simulink model "bp_check_ver1_3"  (R2020b)
settings: Solver=VariableStepAuto  StartTime=0.0  StopTime=20  RelTol=1e-3
undefined symbols (not defined in the file): sigbuilder_block
libraries: simulink x22
settings Model: Creator=HP  LastModifiedBy=HP

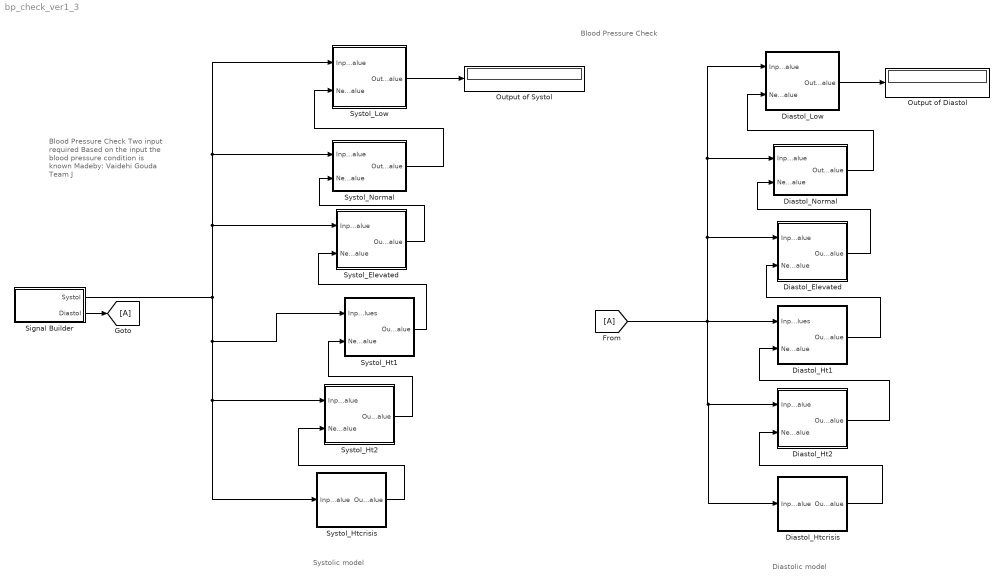
== system bp_check_ver1_3 ==
  note: Systolic model
  note: Blood Pressure Check
      |
      | Two input required
      | Based on the input the blood pressure condition is known
      |
      | Madeby: Vaidehi Gouda
      | Team J
  note: Blood Pressure Check
  note: Diastolic model
  Diastol_Elevated : Subsystem
  Diastol_Ht1 : Subsystem
  Diastol_Ht2 : Subsystem
  Diastol_Htcrisis : Subsystem
  Diastol_Low : Subsystem
  Diastol_Normal : Subsystem
  Output of Diastol : Display
  Output of Systol : Display
  Signal Builder : Subsystem  Tag=STV Subsys  LoadFcn=sigbuilder_block('load');  StartFcn=sigbuilder_block('start');  StopFcn=sigbuilder_block('stop');  ClipboardFcn=sigbuilder_block('clipboard');  mask(Sigbuilder block){tuvar=[0:10]}
      mask help: Simulink:masks:SigbuilderBlock_MD
      mask init:
      | if ~strcmp(get_param(bdroot(gcbh),'SimulationStatus'),'stopped') tuvar = sigbuilder_block('maskInit'); end
      settings: CopyFcn=sigbuilder_block('copy');  DeleteFcn=sigbuilder_block('delete');  ModelCloseFcn=sigbuilder_block('modelClose');  PreSaveFcn=sigbuilder_block('preSave');  PauseFcn=sigbuilder_block('pause');  ContinueFcn=sigbuilder_block('continue');  NameChangeFcn=sigbuilder_block('namechange');  OpenFcn=sigbuilder_block('open',[5.4 30 1141.2 522.6 ]);  CloseFcn=sigbuilder_block('close');
      mask Display: plot(0, 0, 100, 100,[2, 2, 32, 32, 2], [68, 8, 8, 68, 68],[32, 2], [38, 38], [32, 19, 2],[53, 60, 44], [32, 17, 17, 2],[16, 16, 31, 31]);txt = getActiveGroup(gcbh);text(2, 100, txt,'verticalAlignment', 'top');
  Systol_Elevated : Subsystem
  Systol_Ht1 : Subsystem
  Systol_Ht2 : Subsystem
  Systol_Htcrisis : Subsystem
  Systol_Low : Subsystem
  Systol_Normal : Subsystem
  wires:
  Systol_Normal/1(Output_value) -> Systol_Low/2(Next Input value)
  Systol_Elevated/1(Output_value) -> Systol_Normal/2(Next Input value)
  Systol_Ht1/1(Output_value) -> Systol_Elevated/2(Next Input value)
  Systol_Ht2/1(Output_value) -> Systol_Ht1/2(Next Input value)
  Systol_Htcrisis/1(Output_value) -> Systol_Ht2/2(Next Input value)
  Diastol_Htcrisis/1(Output value) -> Diastol_Ht2/2(Next Input value)
  Diastol_Ht2/1(Output_value) -> Diastol_Ht1/2(Next Input value)
  Diastol_Ht1/1(Output_value) -> Diastol_Elevated/2(Next Input value)
  Diastol_Elevated/1(Output value) -> Diastol_Normal/2(Next Input value)
  Diastol_Normal/1(Output_value) -> Diastol_Low/2(Next Input value)
  Diastol_Low/1(Output_value) -> Output of Diastol/1
  Signal Builder/1(Systol) -> Systol_Htcrisis/1(Input value), Systol_Ht2/1(Input value), Systol_Ht1/1(Input values), Systol_Elevated/1(Input value), Systol_Normal/1(Input value), Systol_Low/1(Input_value)
  Systol_Low/1(Output_value) -> Output of Systol/1
  [A] -> Diastol_Elevated/1(Input value), Diastol_Normal/1(Input value), Diastol_Low/1(Input_value), Diastol_Htcrisis/1(Input value), Diastol_Ht2/1(Input value), Diastol_Ht1/1(Input values)
  Signal Builder/2(Diastol) -> [A]

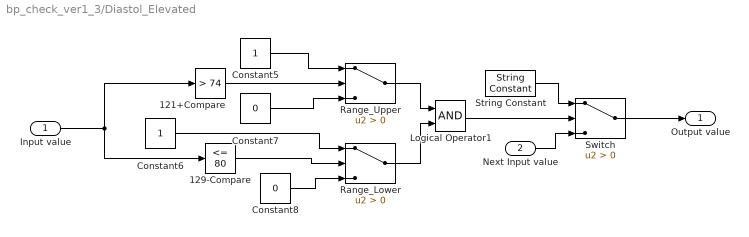
== system bp_check_ver1_3/Diastol_Elevated ==
  Input value : Inport
  Next Input value : Inport  Port=2
  121+Compare : simulink/Logic and Bit Operations/Compare To Constant  relop=>  const=74  OutDataTypeStr=boolean
  129-Compare : simulink/Logic and Bit Operations/Compare To Constant  relop=<=  const=80  OutDataTypeStr=boolean
  Constant5 : Constant
  Constant6 : Constant
  Constant7 : Constant  Value=0
  Constant8 : Constant  Value=0
  Logical Operator1 : Logic  AllPortsSameDT=off  OutDataTypeStr=boolean
  Range_Lower : Switch  Criteria=u2 > Threshold
  Range_Upper : Switch  Criteria=u2 > Threshold
  String Constant : StringConstant  String="\"Eleveted\""
  Switch : Switch  Criteria=u2 > Threshold
  Output value : Outport
  wires:
  Constant7/1 -> Range_Upper/3
  Input value/1 -> 129-Compare/1, 121+Compare/1
  Constant6/1 -> Range_Lower/1
  Constant8/1 -> Range_Lower/3
  Constant5/1 -> Range_Upper/1
  121+Compare/1 -> Range_Upper/2
  Range_Upper/1 -> Logical Operator1/1
  129-Compare/1 -> Range_Lower/2
  Range_Lower/1 -> Logical Operator1/2
  String Constant/1 -> Switch/1
  Logical Operator1/1 -> Switch/2
  Switch/1 -> Output value/1
  Next Input value/1 -> Switch/3

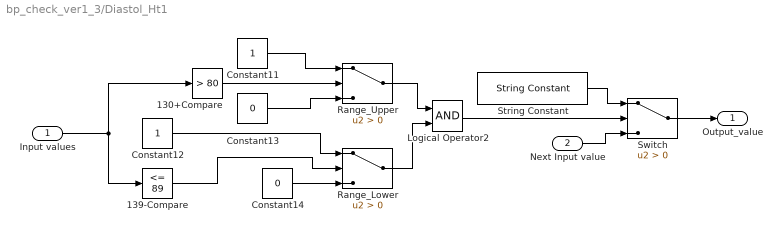
== system bp_check_ver1_3/Diastol_Ht1 ==
  Input values : Inport
  Next Input value : Inport  Port=2
  130+Compare : simulink/Logic and Bit Operations/Compare To Constant  relop=>  const=80  OutDataTypeStr=boolean
  139-Compare : simulink/Logic and Bit Operations/Compare To Constant  relop=<=  const=89  OutDataTypeStr=boolean
  Constant11 : Constant
  Constant12 : Constant
  Constant13 : Constant  Value=0
  Constant14 : Constant  Value=0
  Logical Operator2 : Logic  AllPortsSameDT=off  OutDataTypeStr=boolean
  Range_Lower : Switch  Criteria=u2 > Threshold
  Range_Upper : Switch  Criteria=u2 > Threshold
  String Constant : StringConstant  String="\"Hypertension Stage1\""
  Switch : Switch  Criteria=u2 > Threshold
  Output_value : Outport
  wires:
  Constant13/1 -> Range_Upper/3
  Range_Upper/1 -> Logical Operator2/1
  Range_Lower/1 -> Logical Operator2/2
  139-Compare/1 -> Range_Lower/2
  130+Compare/1 -> Range_Upper/2
  Constant12/1 -> Range_Lower/1
  Constant14/1 -> Range_Lower/3
  Constant11/1 -> Range_Upper/1
  Input values/1 -> 139-Compare/1, 130+Compare/1
  String Constant/1 -> Switch/1
  Logical Operator2/1 -> Switch/2
  Switch/1 -> Output_value/1
  Next Input value/1 -> Switch/3

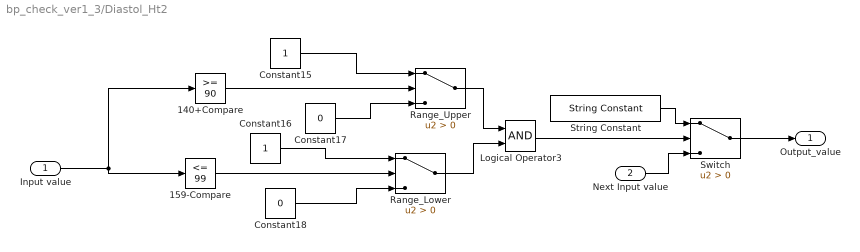
== system bp_check_ver1_3/Diastol_Ht2 ==
  Input value : Inport
  Next Input value : Inport  Port=2
  140+Compare : simulink/Logic and Bit Operations/Compare To Constant  relop=>=  const=90  OutDataTypeStr=boolean
  159-Compare : simulink/Logic and Bit Operations/Compare To Constant  relop=<=  const=99  OutDataTypeStr=boolean
  Constant15 : Constant
  Constant16 : Constant
  Constant17 : Constant  Value=0
  Constant18 : Constant  Value=0
  Logical Operator3 : Logic  AllPortsSameDT=off  OutDataTypeStr=boolean
  Range_Lower : Switch  Criteria=u2 > Threshold
  Range_Upper : Switch  Criteria=u2 > Threshold
  String Constant : StringConstant  String="\"Hypertension Stage2\""
  Switch : Switch  Criteria=u2 > Threshold
  Output_value : Outport
  wires:
  Constant15/1 -> Range_Upper/1
  140+Compare/1 -> Range_Upper/2
  Constant18/1 -> Range_Lower/3
  Range_Lower/1 -> Logical Operator3/2
  Range_Upper/1 -> Logical Operator3/1
  Input value/1 -> 159-Compare/1, 140+Compare/1
  Constant17/1 -> Range_Upper/3
  159-Compare/1 -> Range_Lower/2
  Constant16/1 -> Range_Lower/1
  String Constant/1 -> Switch/1
  Logical Operator3/1 -> Switch/2
  Switch/1 -> Output_value/1
  Next Input value/1 -> Switch/3

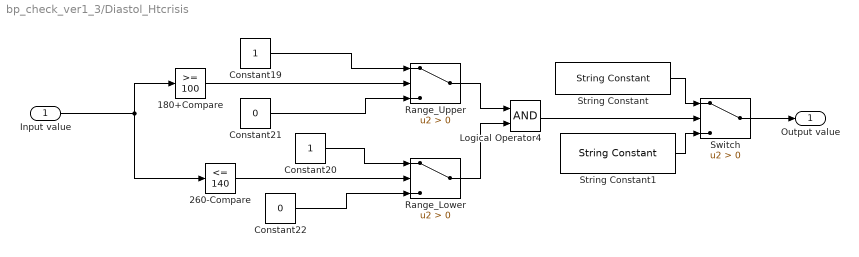
== system bp_check_ver1_3/Diastol_Htcrisis ==
  Input value : Inport
  180+Compare : simulink/Logic and Bit Operations/Compare To Constant  relop=>=  const=100  OutDataTypeStr=boolean
  260-Compare : simulink/Logic and Bit Operations/Compare To Constant  relop=<=  const=140  OutDataTypeStr=boolean
  Constant19 : Constant
  Constant20 : Constant
  Constant21 : Constant  Value=0
  Constant22 : Constant  Value=0
  Logical Operator4 : Logic  AllPortsSameDT=off  OutDataTypeStr=boolean
  Range_Lower : Switch  Criteria=u2 > Threshold
  Range_Upper : Switch  Criteria=u2 > Threshold
  String Constant : StringConstant  String="\"Hypertension crisis\""
  String Constant1 : StringConstant  String="\"Input value not in range\""
  Switch : Switch  Criteria=u2 > Threshold
  Output value : Outport
  wires:
  Input value/1 -> 260-Compare/1, 180+Compare/1
  Constant19/1 -> Range_Upper/1
  Range_Upper/1 -> Logical Operator4/1
  Constant20/1 -> Range_Lower/1
  180+Compare/1 -> Range_Upper/2
  260-Compare/1 -> Range_Lower/2
  Constant22/1 -> Range_Lower/3
  Constant21/1 -> Range_Upper/3
  Range_Lower/1 -> Logical Operator4/2
  String Constant/1 -> Switch/1
  Logical Operator4/1 -> Switch/2
  Switch/1 -> Output value/1
  String Constant1/1 -> Switch/3

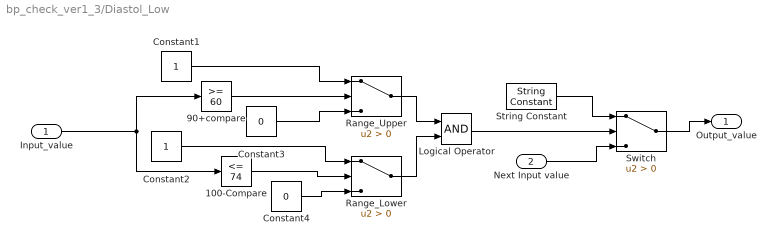
== system bp_check_ver1_3/Diastol_Low ==
  Input_value : Inport
  Next Input value : Inport  Port=2
  100-Compare : simulink/Logic and Bit Operations/Compare To Constant  relop=<=  const=74  OutDataTypeStr=boolean
  90+compare : simulink/Logic and Bit Operations/Compare To Constant  relop=>=  const=60  OutDataTypeStr=boolean
  Constant1 : Constant
  Constant2 : Constant
  Constant3 : Constant  Value=0
  Constant4 : Constant  Value=0
  Logical Operator : Logic  AllPortsSameDT=off  OutDataTypeStr=boolean
  Range_Lower : Switch  Criteria=u2 > Threshold
  Range_Upper : Switch  Criteria=u2 > Threshold
  String Constant : StringConstant  String="\"Low\""
  Switch : Switch  Criteria=u2 > Threshold
  Output_value : Outport
  wires:
  Constant2/1 -> Range_Lower/1
  Constant4/1 -> Range_Lower/3
  90+compare/1 -> Range_Upper/2
  100-Compare/1 -> Range_Lower/2
  Range_Upper/1 -> Logical Operator/1
  Constant1/1 -> Range_Upper/1
  Range_Lower/1 -> Logical Operator/2
  Input_value/1 -> 90+compare/1, 100-Compare/1
  Constant3/1 -> Range_Upper/3
  String Constant/1 -> Switch/1
  Logical Operator/1 -> Switch/2
  Switch/1 -> Output_value/1
  Next Input value/1 -> Switch/3

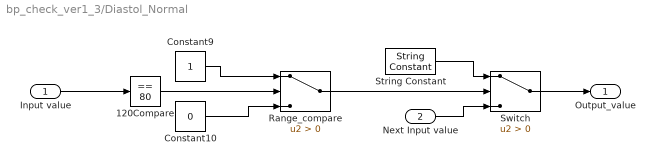
== system bp_check_ver1_3/Diastol_Normal ==
  Input value : Inport
  Next Input value : Inport  Port=2
  120Compare : simulink/Logic and Bit Operations/Compare To Constant  relop===  const=80  OutDataTypeStr=boolean
  Constant10 : Constant  Value=0
  Constant9 : Constant
  Range_compare : Switch  Criteria=u2 > Threshold
  String Constant : StringConstant  String="\"Normal\""
  Switch : Switch  Criteria=u2 > Threshold
  Output_value : Outport
  wires:
  Constant10/1 -> Range_compare/3
  Input value/1 -> 120Compare/1
  120Compare/1 -> Range_compare/2
  Constant9/1 -> Range_compare/1
  String Constant/1 -> Switch/1
  Range_compare/1 -> Switch/2
  Switch/1 -> Output_value/1
  Next Input value/1 -> Switch/3

== system bp_check_ver1_3/Signal Builder ==
  Demux : Demux  Tag=STV Demux  Outputs=2
      settings: DisplayOption=none
  FromWs : FromWorkspace  Tag=STV FromWs  VariableName=tuvar
      SigBuilderData=|
      | common.afterFinalStr = 'Extrapolate'
      | common.sampleTime = 0
      | dataSet.timeRange = [0 2]
      | dataSet.name = 'Sheet1'
      | sbobj.Name = 'Signal Builder'
      | sbobj.Groups.Name = 'Sheet1'
      | sbobj.Groups.Signals(1).Name = 'Systol'
      | sbobj.Groups.Signals(1).XData = [0 0.1 0.2 0.3 0.4 0.5 0.6 0.7 0.8 0.9 1 1.1 1.2 1.3 1.4 1.5 1.6 1.7 1.8 1.9 2]
      | sbobj.Groups.Signals(1).YData = [91 145 132 130 136 140 156 180 95 100 105 102 148 196 142 158 136 135 129 96 109]
      | sbobj.Groups.Signals(2).Name = 'Diastol'
      | sbobj.Groups.Signals(2).XData = [0 0.1 0.2 0.3 0.4 0.5 0.6 0.7 0.8 0.9 1 1.1 1.2 1.3 1.4 1.5 1.6 1.7 1.8 1.9 2]
      | sbobj.Groups.Signals(2).YData = [60 97 84 89 84 90 97 127 67 64 65 64 94 135 98 99 82 84 76 63 70]
      | sbobj.Groups.TimeRange = [0 2]
  Systol : Outport  Tag=STV Outport
  Diastol : Outport  Tag=STV Outport  Port=2
  wires:
  Demux/1 -> Systol/1
  FromWs/1 -> Demux/1
  Demux/2 -> Diastol/1

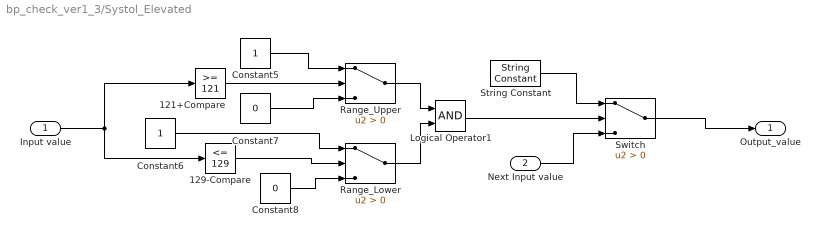
== system bp_check_ver1_3/Systol_Elevated ==
  Input value : Inport
  Next Input value : Inport  Port=2
  121+Compare : simulink/Logic and Bit Operations/Compare To Constant  relop=>=  const=121  OutDataTypeStr=boolean
  129-Compare : simulink/Logic and Bit Operations/Compare To Constant  relop=<=  const=129  OutDataTypeStr=boolean
  Constant5 : Constant
  Constant6 : Constant
  Constant7 : Constant  Value=0
  Constant8 : Constant  Value=0
  Logical Operator1 : Logic  AllPortsSameDT=off  OutDataTypeStr=boolean
  Range_Lower : Switch  Criteria=u2 > Threshold
  Range_Upper : Switch  Criteria=u2 > Threshold
  String Constant : StringConstant  String="\"Elevated\""
  Switch : Switch  Criteria=u2 > Threshold
  Output_value : Outport
  wires:
  Range_Lower/1 -> Logical Operator1/2
  129-Compare/1 -> Range_Lower/2
  Range_Upper/1 -> Logical Operator1/1
  121+Compare/1 -> Range_Upper/2
  Constant5/1 -> Range_Upper/1
  Constant8/1 -> Range_Lower/3
  Constant6/1 -> Range_Lower/1
  Input value/1 -> 121+Compare/1, 129-Compare/1
  Constant7/1 -> Range_Upper/3
  String Constant/1 -> Switch/1
  Logical Operator1/1 -> Switch/2
  Switch/1 -> Output_value/1
  Next Input value/1 -> Switch/3

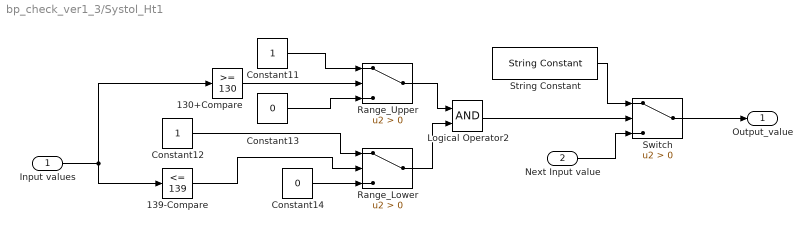
== system bp_check_ver1_3/Systol_Ht1 ==
  Input values : Inport
  Next Input value : Inport  Port=2
  130+Compare : simulink/Logic and Bit Operations/Compare To Constant  relop=>=  const=130  OutDataTypeStr=boolean
  139-Compare : simulink/Logic and Bit Operations/Compare To Constant  relop=<=  const=139  OutDataTypeStr=boolean
  Constant11 : Constant
  Constant12 : Constant
  Constant13 : Constant  Value=0
  Constant14 : Constant  Value=0
  Logical Operator2 : Logic  AllPortsSameDT=off  OutDataTypeStr=boolean
  Range_Lower : Switch  Criteria=u2 > Threshold
  Range_Upper : Switch  Criteria=u2 > Threshold
  String Constant : StringConstant  String="\"Hypertension Stage1\""
  Switch : Switch  Criteria=u2 > Threshold
  Output_value : Outport
  wires:
  Input values/1 -> 139-Compare/1, 130+Compare/1
  Constant11/1 -> Range_Upper/1
  Constant14/1 -> Range_Lower/3
  Constant12/1 -> Range_Lower/1
  130+Compare/1 -> Range_Upper/2
  139-Compare/1 -> Range_Lower/2
  Range_Lower/1 -> Logical Operator2/2
  Range_Upper/1 -> Logical Operator2/1
  Constant13/1 -> Range_Upper/3
  String Constant/1 -> Switch/1
  Logical Operator2/1 -> Switch/2
  Switch/1 -> Output_value/1
  Next Input value/1 -> Switch/3

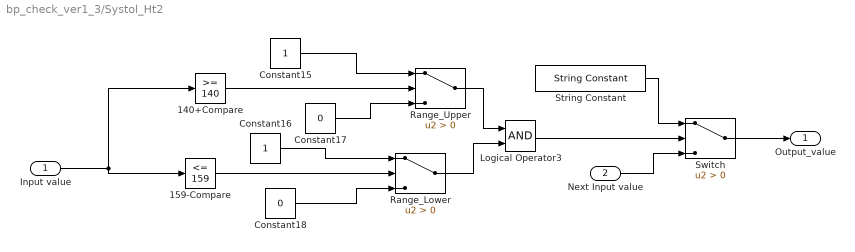
== system bp_check_ver1_3/Systol_Ht2 ==
  Input value : Inport
  Next Input value : Inport  Port=2
  140+Compare : simulink/Logic and Bit Operations/Compare To Constant  relop=>=  const=140  OutDataTypeStr=boolean
  159-Compare : simulink/Logic and Bit Operations/Compare To Constant  relop=<=  const=159  OutDataTypeStr=boolean
  Constant15 : Constant
  Constant16 : Constant
  Constant17 : Constant  Value=0
  Constant18 : Constant  Value=0
  Logical Operator3 : Logic  AllPortsSameDT=off  OutDataTypeStr=boolean
  Range_Lower : Switch  Criteria=u2 > Threshold
  Range_Upper : Switch  Criteria=u2 > Threshold
  String Constant : StringConstant  String="\"Hypertension Stage2\""
  Switch : Switch  Criteria=u2 > Threshold
  Output_value : Outport
  wires:
  Constant16/1 -> Range_Lower/1
  159-Compare/1 -> Range_Lower/2
  Constant17/1 -> Range_Upper/3
  Input value/1 -> 140+Compare/1, 159-Compare/1
  Range_Upper/1 -> Logical Operator3/1
  Range_Lower/1 -> Logical Operator3/2
  Constant18/1 -> Range_Lower/3
  140+Compare/1 -> Range_Upper/2
  Constant15/1 -> Range_Upper/1
  String Constant/1 -> Switch/1
  Logical Operator3/1 -> Switch/2
  Switch/1 -> Output_value/1
  Next Input value/1 -> Switch/3

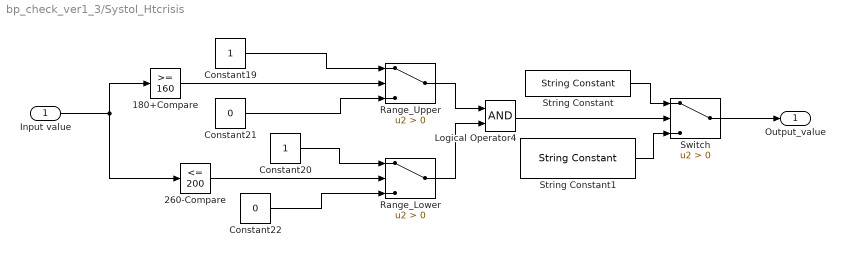
== system bp_check_ver1_3/Systol_Htcrisis ==
  Input value : Inport
  180+Compare : simulink/Logic and Bit Operations/Compare To Constant  relop=>=  const=160  OutDataTypeStr=boolean
  260-Compare : simulink/Logic and Bit Operations/Compare To Constant  relop=<=  const=200  OutDataTypeStr=boolean
  Constant19 : Constant
  Constant20 : Constant
  Constant21 : Constant  Value=0
  Constant22 : Constant  Value=0
  Logical Operator4 : Logic  AllPortsSameDT=off  OutDataTypeStr=boolean
  Range_Lower : Switch  Criteria=u2 > Threshold
  Range_Upper : Switch  Criteria=u2 > Threshold
  String Constant : StringConstant  String="\"Hypertension crisis\""
  String Constant1 : StringConstant  String="\"Input value not in range\""
  Switch : Switch  Criteria=u2 > Threshold
  Output_value : Outport
  wires:
  Range_Lower/1 -> Logical Operator4/2
  Constant21/1 -> Range_Upper/3
  Constant22/1 -> Range_Lower/3
  260-Compare/1 -> Range_Lower/2
  180+Compare/1 -> Range_Upper/2
  Constant20/1 -> Range_Lower/1
  Range_Upper/1 -> Logical Operator4/1
  Constant19/1 -> Range_Upper/1
  Input value/1 -> 180+Compare/1, 260-Compare/1
  String Constant/1 -> Switch/1
  Logical Operator4/1 -> Switch/2
  Switch/1 -> Output_value/1
  String Constant1/1 -> Switch/3

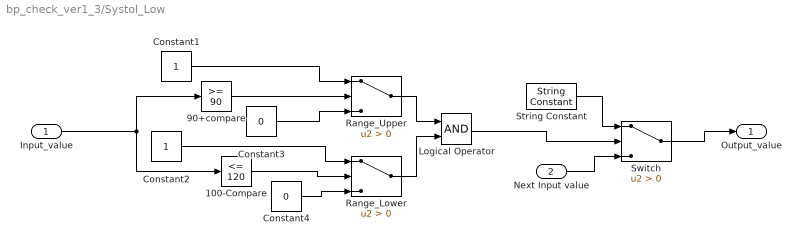
== system bp_check_ver1_3/Systol_Low ==
  Input_value : Inport
  Next Input value : Inport  Port=2
  100-Compare : simulink/Logic and Bit Operations/Compare To Constant  relop=<=  const=120  OutDataTypeStr=boolean
  90+compare : simulink/Logic and Bit Operations/Compare To Constant  relop=>=  const=90  OutDataTypeStr=boolean
  Constant1 : Constant
  Constant2 : Constant
  Constant3 : Constant  Value=0
  Constant4 : Constant  Value=0
  Logical Operator : Logic  AllPortsSameDT=off  OutDataTypeStr=boolean
  Range_Lower : Switch  Criteria=u2 > Threshold
  Range_Upper : Switch  Criteria=u2 > Threshold
  String Constant : StringConstant  String="\"Low\""
  Switch : Switch  Criteria=u2 > Threshold
  Output_value : Outport
  wires:
  Logical Operator/1 -> Switch/2
  Constant3/1 -> Range_Upper/3
  Input_value/1 -> 100-Compare/1, 90+compare/1
  Range_Lower/1 -> Logical Operator/2
  Constant1/1 -> Range_Upper/1
  Range_Upper/1 -> Logical Operator/1
  100-Compare/1 -> Range_Lower/2
  90+compare/1 -> Range_Upper/2
  Constant4/1 -> Range_Lower/3
  Constant2/1 -> Range_Lower/1
  String Constant/1 -> Switch/1
  Switch/1 -> Output_value/1
  Next Input value/1 -> Switch/3

== system bp_check_ver1_3/Systol_Normal ==
  Input value : Inport
  Next Input value : Inport  Port=2
  120Compare : simulink/Logic and Bit Operations/Compare To Constant  relop===  const=120  OutDataTypeStr=boolean
  Constant10 : Constant  Value=0
  Constant9 : Constant
  Range_compare : Switch  Criteria=u2 > Threshold
  String Constant : StringConstant  String="\"Normal\""
  Switch : Switch  Criteria=u2 > Threshold
  Output_value : Outport
  wires:
  Constant9/1 -> Range_compare/1
  120Compare/1 -> Range_compare/2
  Input value/1 -> 120Compare/1
  Constant10/1 -> Range_compare/3
  String Constant/1 -> Switch/1
  Range_compare/1 -> Switch/2
  Switch/1 -> Output_value/1
  Next Input value/1 -> Switch/3
